simulink model "LatcontrollerSim"  (R2017a)
settings: Solver=VariableStepAuto  StartTime=0.0  StopTime=20  RelTol=1e-3
values from neighbouring files (symbols this model uses):
  a1 = 1*1    (= 1)    [Latcontroller.m]
  a2 = 0.001*1    (= 0.001)    [Latcontroller.m]
  den = [den1 den2 den3]    [Latcontroller.m]
  initial = [1 0 0/57.3 0]    [Latcontroller.m]
  Kc = lqr(matrix_a_,matrix_b_,matrix_q_,matrix_r_)*Kcp    [Latcontroller.m]
  Ki = 0.2    [Latcontroller.m]
  Ksteer = 1    [Latcontroller.m]
  matrix_a_ = zeros(basic_state_size_, basic_state_size_)    [Latcontroller.m]
  matrix_b_ = zeros(basic_state_size_, 1)    [Latcontroller.m]
  num = [num1 num2 num3]    [Latcontroller.m]
  steer0 = -1/57.3    (= -0.0174520069808)    [Latcontroller.m]
  steerdelay = 0.4*1    (= 0.4)    [Latcontroller.m]
  Tc = 0.1    [Latcontroller.m]
  TFK = ts    (= 0.01)    [Latcontroller.m]
  Tnavigation = 0.005    [Latcontroller.m]
  Tsteer = 0.2*1    (= 0.2)    [Latcontroller.m]
  Zc = 0/57.3    (= 0)    [Latcontroller.m]
settings Model: Creator=baowen  LastModifiedBy=baowen

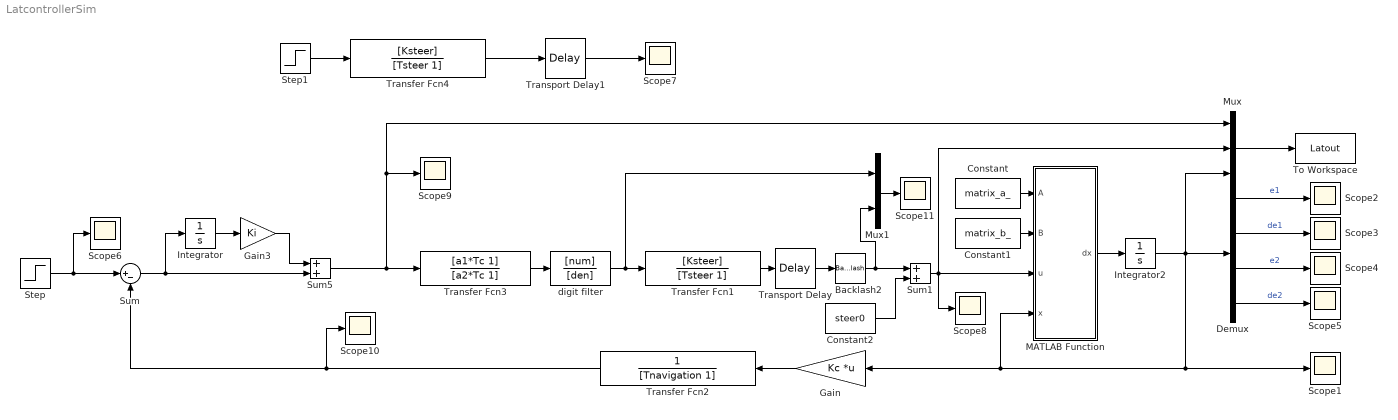
== system LatcontrollerSim ==
  Backlash2 : Backlash  BacklashWidth=backlash
  Constant : Constant  Value=matrix_a_
  Constant1 : Constant  Value=matrix_b_
  Constant2 : Constant  Value=steer0
  Demux : Demux
  Gain : Gain  Gain=Kc  Multiplication=Matrix(K*u)
  Gain3 : Gain  Gain=Ki
  Integrator : Integrator
  Integrator2 : Integrator  InitialCondition=initial
  MATLAB Function : MATLAB Function  TreatAsAtomicUnit=on
  Mux : Mux  Inputs=3
  Mux1 : Mux  Inputs=2
  Scope{1..11} (11 alike) : Scope
  Step : Step  Time=0  After=Zc  SampleTime=0
  Step1 : Step  Time=0  SampleTime=0
  Sum : Sum  Inputs=|+-
  Sum1 : Sum
  Sum5 : Sum
  To Workspace : ToWorkspace  VariableName=Latout  SaveFormat=Timeseries  SampleTime=TFK
  Transfer Fcn1 : TransferFcn  Numerator=[Ksteer]  Denominator=[Tsteer 1]
  Transfer Fcn2 : TransferFcn  Denominator=[Tnavigation 1]
  Transfer Fcn3 : TransferFcn  Numerator=[a1*Tc 1]  Denominator=[a2*Tc 1]
  Transfer Fcn4 : TransferFcn  Numerator=[Ksteer]  Denominator=[Tsteer 1]
  Transport Delay : TransportDelay  DelayTime=steerdelay
  Transport Delay1 : TransportDelay  DelayTime=steerdelay
  digit filter : TransferFcn  Numerator=[num]  Denominator=[den]
  wires:
  Step/1 -> Scope6/1, Sum/1
  Constant/1 -> MATLAB Function/1(A)
  Constant1/1 -> MATLAB Function/2(B)
  Demux/1 -> Scope2/1  "e1"
  Demux/2 -> Scope3/1  "de1"
  Demux/4 -> Scope5/1  "de2"
  Demux/3 -> Scope4/1  "e2"
  MATLAB Function/1(dx) -> Integrator2/1
  Gain/1 -> Transfer Fcn2/1
  Mux/1 -> To Workspace/1
  Integrator2/1 -> Scope1/1, Gain/1, MATLAB Function/4(x), Demux/1, Mux/3
  Transfer Fcn2/1 -> Scope10/1, Sum/2
  Transfer Fcn3/1 -> digit filter/1
  Transfer Fcn4/1 -> Transport Delay1/1
  Transport Delay1/1 -> Scope7/1
  Step1/1 -> Transfer Fcn4/1
  Transport Delay/1 -> Backlash2/1
  Sum1/1 -> Scope8/1, Mux/2, MATLAB Function/3(u)
  Sum5/1 -> Transfer Fcn3/1, Scope9/1, Mux/1
  Sum/1 -> Integrator/1, Sum5/2
  Integrator/1 -> Gain3/1
  Gain3/1 -> Sum5/1
  Transfer Fcn1/1 -> Transport Delay/1
  Mux1/1 -> Scope11/1
  digit filter/1 -> Transfer Fcn1/1, Mux1/1
  Backlash2/1 -> Mux1/2, Sum1/1
  Constant2/1 -> Sum1/2

== matlab function LatcontrollerSim/MATLAB Function ==
  data: A input; B input; u input; dx output; x input
function dx  = fcn(A,B,u,x)

% x=x+[0;0;0;0];
dx= A*x+B*u;
